simulink model "sim_model"  (R2021a)
settings: Solver=ode4  StartTime=0.0  StopTime=1000  FixedStep=1e-4  RelTol=1e-3
values from neighbouring files (symbols this model uses):
  c_e = 300    [config.m]
  c_M = 300    [config.m]
  F_N = i_VN * w    (= 19465.0205761)    [config.m]
  Fi_N = 0.005    [config.m]
  i_GN = i_N + i_VN    (= 32.2633744856)    [config.m]
  i_N = 30    [config.m]
  J = 0.12    [config.m]
  L_YA = 0.02    [config.m]
  M_VN = 50    [config.m]
  omega_N = 100    [config.m]
  p = [-0.0014 0.1628 -0.4707 0.4731 -0.0316 0]    [config.m]
  R_0N = 4    [config.m]
  r_V = 97.2    [config.m]
  r_YA = 1.39    [config.m]
  w = 8600    [config.m]    (also in eiler.m = x)
settings Model: Creator=Asik  LastModifiedBy=Nikitos
settings SolverCC: AlgebraicLoopSolver=TrustRegion
settings DebuggingCC: SFMachineParentedDataDiag=warning
settings SFSimCC: CustomCodeUndefinedFunction=UseInterfaceOnly

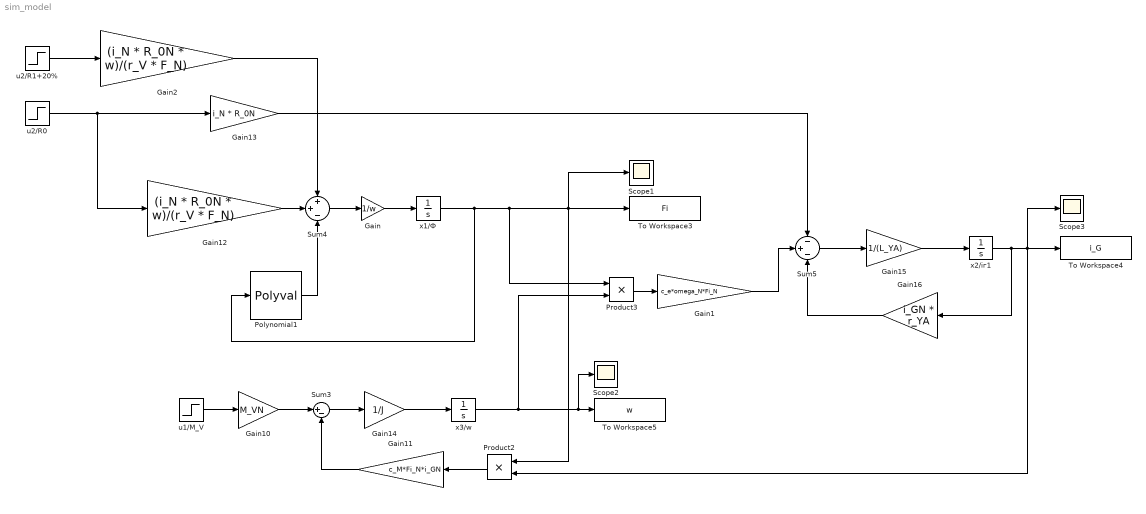
== system sim_model ==
  Gain : Gain  Gain=1/w
  Gain1 : Gain  Gain=c_e*omega_N*Fi_N
  Gain10 : Gain  Gain=M_VN
  Gain11 : Gain  Gain=c_M*Fi_N*i_GN
  Gain12 : Gain  Gain=(i_N * R_0N * w)/(r_V * F_N)
  Gain13 : Gain  Gain=i_N * R_0N
  Gain14 : Gain  Gain=1/J
  Gain15 : Gain  Gain=1/(L_YA)
  Gain16 : Gain  Gain=i_GN * r_YA
  Gain2 : Gain  Gain=(i_N * R_0N * w)/(r_V * F_N)
  Polynomial1 : Polyval  Coefs=p
  Product2 : Product
  Product3 : Product
  Scope1 : Scope
  Scope2 : Scope
  Scope3 : Scope
  Sum3 : Sum  Inputs=|+-
  Sum4 : Sum  Inputs=++-
  Sum5 : Sum  Inputs=-+-
  To Workspace3 : ToWorkspace  VariableName=Fi  SaveFormat=Timeseries  SampleTime=-1
  To Workspace4 : ToWorkspace  VariableName=i_G  SaveFormat=Timeseries  SampleTime=-1
  To Workspace5 : ToWorkspace  VariableName=w  SaveFormat=Timeseries  SampleTime=-1
  u1/M_V : Step  Time=0  SampleTime=0
  u2/R0 : Step  Time=0  SampleTime=0
  u2/R1+20% : Step  Time=100000  SampleTime=0
  x1/Ф : Integrator
  x2/iг1 : Integrator
  x3/w : Integrator
  wires:
  u1/M_V/1 -> Gain10/1
  Gain10/1 -> Sum3/1
  Gain11/1 -> Sum3/2
  Product2/1 -> Gain11/1
  x1/Ф/1 -> Polynomial1/1, Product3/1, Scope1/1, Product2/1, To Workspace3/1
  u2/R0/1 -> Gain12/1, Gain13/1
  Gain13/1 -> Sum5/1
  Sum3/1 -> Gain14/1
  Gain14/1 -> x3/w/1
  Gain15/1 -> x2/iг1/1
  x2/iг1/1 -> Gain16/1, Product2/2, Scope3/1, To Workspace4/1
  Gain16/1 -> Sum5/3
  x3/w/1 -> Scope2/1, To Workspace5/1, Product3/2
  Gain/1 -> x1/Ф/1
  Sum4/1 -> Gain/1
  Product3/1 -> Gain1/1
  Gain1/1 -> Sum5/2
  Polynomial1/1 -> Sum4/3
  Gain12/1 -> Sum4/2
  u2/R1+20%/1 -> Gain2/1
  Gain2/1 -> Sum4/1
  Sum5/1 -> Gain15/1
